simulink model "A5_Fahrzeugmodell_linear"  (R2017b)
settings: Solver=ode45  StartTime=0.0  StopTime=500  MaxStep=1E-2  RelTol=1e-3  EnableMultiTasking=on
values from neighbouring files (symbols this model uses):
  cL = 20    [A5_Konstanten.m]
  m = 1000    [A5_Konstanten.m]    (also in Model_1_Konstanten.m)
undefined symbols (not defined in the file or in its folder): sigbuilder_block
settings Model: Creator=jbaur  LastModifiedBy=jbaur
settings DataIOCC: ExternalInput=X1  SaveFormat=StructureWithTime  SignalLoggingName=sigsOut
settings OptimizationCC: ExpressionDepthLimit=2147483647  InitFltsAndDblsToZero=on  LifeSpan=inf
settings DebuggingCC: SaveWithParameterizedLinksMsg=none  SignalResolutionControl=TryResolveAllWithWarning  MultiTaskDSMMsg=warning  MultiTaskCondExecSysMsg=none  StateNameClashWarn=warning  SFUnexpectedBacktrackingDiag=warning  SFNoUnconditionalDefaultTransitionDiag=warning  SFExecutionAtInitializationDiag=none
settings HardwareCC: ProdBitPerPointer=32  ProdBitPerSizeT=32  ProdBitPerPtrDiffT=32  ProdLargestAtomicFloat=None  ProdIntDivRoundTo=Undefined  ProdEndianess=Unspecified  ProdWordSize=32  ProdHWDeviceType=32-bit Generic  TargetUnknown=on
settings ModelReferenceCC: PropagateSignalLabelsOutOfModel=off
settings CodeAppCC: StateflowObjectComments=on
settings GRTTargetCC: TargetFcnLib=ansi_tfl_tmw.mat  TargetLangStandard=C89/C90 (ANSI)  ModelReferenceCompliant=off  GeneratePreprocessorConditionals=Disable all  CombineOutputUpdateFcns=off  MatFileLogging=off  GRTInterface=on
settings ConfigComp: CovMetricSettings=dw  CovHtmlReporting=on  CovSaveCumulativeToWorkspaceVar=on  CovSaveSingleToWorkspaceVar=on  CovExternalEMLEnable=off  CovSFcnEnable=off

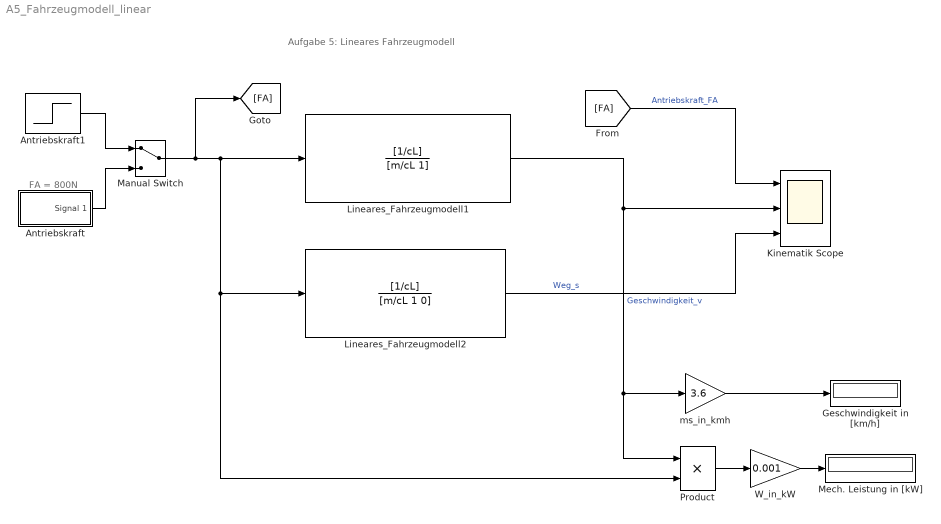
== system A5_Fahrzeugmodell_linear ==
  note: Aufgabe 5: Lineares Fahrzeugmodell
  note: FA = 800N
  Antriebskraft : Subsystem  Tag=STV Subsys  LoadFcn=sigbuilder_block('load');  StartFcn=sigbuilder_block('start');  StopFcn=sigbuilder_block('stop');  ClipboardFcn=sigbuilder_block('clipboard');  mask(Sigbuilder block){tuvar=[0:10]}
      mask help: Sigbuilder GUI
      mask init:
      | if ~strcmp(get_param(bdroot(gcbh),'SimulationStatus'),'stopped') tuvar = sigbuilder_block('maskInit'); end
      settings: CopyFcn=sigbuilder_block('copy');  DeleteFcn=sigbuilder_block('delete');  ModelCloseFcn=sigbuilder_block('modelClose');  PreSaveFcn=sigbuilder_block('preSave');  PauseFcn=sigbuilder_block('pause')  ContinueFcn=sigbuilder_block('continue')  NameChangeFcn=sigbuilder_block('namechange');  OpenFcn=sigbuilder_block('open',[174.75 101.25 550.5 363.75 ]);  CloseFcn=sigbuilder_block('close');
      mask Display: plot(0, 0, 100, 100,[2, 2, 32, 32, 2], [68, 8, 8, 68, 68],[32, 2], [38, 38], [32, 19, 2],[53, 60, 44], [32, 17, 17, 2],[16, 16, 31, 31]);txt = getActiveGroup(gcbh);text(2, 100, txt,'verticalAlignment', 'top');
  Antriebskraft1 : Step  After=800  SampleTime=0
  Geschwindigkeit in [km/h] : Display
  Kinematik Scope : Scope  NumInputPorts=3
  Lineares_Fahrzeugmodell1 : TransferFcn  Numerator=[1/cL]  Denominator=[m/cL 1]
  Lineares_Fahrzeugmodell2 : TransferFcn  Numerator=[1/cL]  Denominator=[m/cL 1 0]
  Manual Switch : ManualSwitch
  Mech. Leistung in [kW] : Display
  Product : Product  RndMeth=Zero
  W_in_kW : Gain  Gain=0.001
  ms_in_kmh : Gain  Gain=3.6
  wires:
  Lineares_Fahrzeugmodell1/1 -> Product/1, ms_in_kmh/1, Kinematik Scope/2  "Geschwindigkeit_v"
  Lineares_Fahrzeugmodell2/1 -> Kinematik Scope/3  "Weg_s"
  Manual Switch/1 -> [FA], Lineares_Fahrzeugmodell1/1, Lineares_Fahrzeugmodell2/1, Product/2
  [FA] -> Kinematik Scope/1  "Antriebskraft_FA"
  Antriebskraft/1(Signal 1) -> Manual Switch/2
  Antriebskraft1/1 -> Manual Switch/1
  ms_in_kmh/1 -> Geschwindigkeit in [km/h]/1
  Product/1 -> W_in_kW/1
  W_in_kW/1 -> Mech. Leistung in [kW]/1

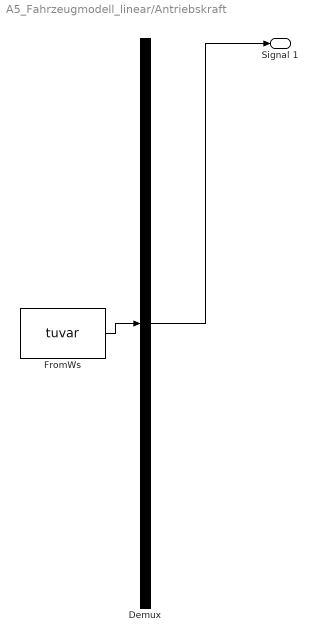
== system A5_Fahrzeugmodell_linear/Antriebskraft ==
  Demux : Demux  Tag=STV Demux  Outputs=1
  FromWs : FromWorkspace  Tag=STV FromWs  VariableName=tuvar  SampleTime=0
      SigBuilderData=|
      | common.afterFinalStr = 'Extrapolate'
      | common.sampleTime = 0
      | dataSet.timeRange = [0 200]
      | dataSet.name = 'Group 1'
      | sbobj.Groups.Name = 'Group 1'
      | sbobj.Groups.Signals.Name = 'Signal 1'
      | sbobj.Groups.Signals.XData = [0 4 4 100 100 200]
      | sbobj.Groups.Signals.YData = [0 0 800 800 0 0]
      | sbobj.Groups.TimeRange = [0 200]
  Signal 1 : Outport  Tag=STV Outport
  wires:
  Demux/1 -> Signal 1/1
  FromWs/1 -> Demux/1
